simulink model "GolfSwing3D_SimscapePhysicalInterfaceSwitching"  (R2024b)
settings: Solver=VariableStepAuto  StartTime=0.0  StopTime=StopTime  MaxStep=0.001  RelTol=1e-3
model workspace: external: MAT-File 3DModelInputs.mat (data not in the file)
undefined symbols (not defined in the file): GripStrength, KillswitchFinalValue, KillswitchInitialValue, KillswitchStepTime, LeftLowerArmLength, PlaneTilt, RightLowerArmLength, UpperTorsoLength, X, Y, Z
libraries: nesl_utility x363, sm_lib x137, matrix_library x11, fl_lib x8, simulink x1
(part 10 of 13)

== system GolfSwing3D_SimscapePhysicalInterfaceSwitching/Left Elbow Joint/Revolute Joint/Subsystem ==
  note: Kinetic Enabled Subsystem
  Angular Velocity (rad/s) : Inport
  Enable : EnablePort
  Constant2 : Constant  Value=10
  Ideal Torque Sensor : fl_lib/Mechanical/Mechanical Sensors/Ideal Torque Sensor
  Ideal Torque Source : fl_lib/Mechanical/Mechanical Sources/Ideal Torque Source
  Mechanical Rotational Reference : fl_lib/Mechanical/Rotational Elements/Mechanical Rotational Reference
  PS-Simulink Converter : nesl_utility/PS-Simulink Converter  PhysicalDomain=network_engine_domain  SubClassName=ps_output  LeftPortType=input  RightPortType=output  PseudoPeriodic=off  Frequencies=[]  VectorFormat=inherit  Unit=inherit  AffineConversion=off
  Rotational Multibody Interface1 : fl_lib/Mechanical/Multibody Interfaces/Rotational Multibody Interface
  Simulink-PS Converter : nesl_utility/Simulink-PS Converter  PhysicalDomain=network_engine_domain  SubClassName=ps_input  LeftPortType=input  RightPortType=output  PseudoPeriodic=off  Frequencies=[]  NoiseDistribution=none  NoiseParameters=[]  Unit=rad/s  AffineConversion=off  FilteringAndDerivatives=provide  SimscapeFilterOrder=1  InputFilterTimeConstant=0.001  UdotUserProvided=0
  Simulink-PS Converter2 : nesl_utility/Simulink-PS Converter  PhysicalDomain=network_engine_domain  SubClassName=ps_input  LeftPortType=input  RightPortType=output  PseudoPeriodic=off  Frequencies=[]  NoiseDistribution=none  NoiseParameters=[]  Unit=1  AffineConversion=off  FilteringAndDerivatives=provide  SimscapeFilterOrder=1  InputFilterTimeConstant=0.001  UdotUserProvided=0
  Solver Configuration : nesl_utility/Solver Configuration  PhysicalDomain=network_engine_domain  SubClassName=solver  LeftPortType=input  RightPortType=generic  Tones=[]  Harmonics=[]  SimulateNoise=off  Profile=off  UseLocalSampling=off  EnableSwitchedLinearOptims=on  FrequencyDomain=off  UseCCode=off  RelTol=0.001  AbsTol=0.001  MinStep=1e-09  ToWorkspace=off  RevertToSquareIcSolve=off  NumHomotopyIterations=100  PhasorMode=off  PhasorModeNumHarmonics=1  ConsistencySolver=NEWTON_XTOL_AFTER_FTOL  IndexReductionMethod=DerivativeReplacement  DoDC=off  ResidualTolerance=1e-09  ConsistencyTolSource=GLOBAL  ConsistencyAbsTol=0.001  ConsistencyRelTol=0.001  ConsistencyTolFactor=0.001  UseLocalSolver=off  LocalSolverChoice=NE_BACKWARD_EULER_ADVANCER  ResolveIndetEquations=on  FunctionEvalNumThread=1  LocalSolverSampleTime=0.001  DoFixedCost=off  MaxNonlinIter=3  MaxModeIter=2  ComputeImpulses=off  ImpulseIterations=2  LinearAlgebra=auto  LinearAlgebraNumThread=0  EquationFormulation=NE_TIME_EF  DelaysMemoryBudget=1024  AutomaticFiltering=on  FilteringTimeConstant=0.001  PartitionStorageMethod=AS_NEEDED  PartitionMemoryBudget=1024  PartitionMethod=ROBUST  MultibodyUseLocalSolver=off  MultibodyLocalSolverChoice=ODE1  MultibodyLocalSolverSampleTime=0.001
  Torque (Nm) : Outport
  wires:
  Constant2/1 -> Simulink-PS Converter2/1
  PS-Simulink Converter/1 -> Torque (Nm)/1
  Angular Velocity (rad/s)/1 -> Simulink-PS Converter/1
  connections:
  Ideal Torque Sensor/RConn1 -- Rotational Multibody Interface1/RConn2
  Mechanical Rotational Reference/LConn1 -- Ideal Torque Source/RConn2 -- Solver Configuration/RConn1 -- Rotational Multibody Interface1/LConn2
  Rotational Multibody Interface1/LConn1 -- PS-Simulink Converter/LConn1
  Ideal Torque Source/LConn1 -- Ideal Torque Sensor/LConn1
  Simulink-PS Converter2/RConn1 -- Ideal Torque Source/RConn1
  Rotational Multibody Interface1/RConn1 -- Simulink-PS Converter/RConn1

== system GolfSwing3D_SimscapePhysicalInterfaceSwitching/Left Forearm/Left Forearm/LF Kinematically Driven ==
  Kinematically Driven LF : sm_lib/Joints/Revolute Joint  JointMode=Normal  CompositeWrenchDir=BaseOnFollower  CompositeWrenchFrame=FollowerFrame  SenseConstraintForce=off  SenseConstraintTorque=off  SenseTotalForce=off  SenseTotalTorque=on  PositionTargetSpecify=off  PositionTargetPriority=Low  PositionTargetValue=LFStartPosition  PositionTargetValueUnits=deg  VelocityTargetSpecify=off  VelocityTargetPriority=Low  VelocityTargetValue=LFStartVelocity  VelocityTargetValueUnits=deg/s  EquilibriumPosition=0  EquilibriumPositionUnits=deg  SpringStiffness=0  SpringStiffnessUnits=N*m/deg  DampingCoefficient=0  DampingCoefficientUnits=N*m/(deg/s)  LowerLimitSpecify=off  LowerLimitBound=0  LowerLimitBoundUnits=deg  LowerLimitStiffness=50  LowerLimitStiffnessUnits=N*m/deg  LowerLimitDamping=10  LowerLimitDampingUnits=N*m/(deg/s)  LowerLimitTransitionRegionWidth=0.1  LowerLimitTransitionRegionWidthUnits=deg  UpperLimitSpecify=off  UpperLimitBound=75  UpperLimitBoundUnits=deg  UpperLimitStiffness=50  UpperLimitStiffnessUnits=N*m/deg  UpperLimitDamping=10  UpperLimitDampingUnits=N*m/(deg/s)  UpperLimitTransitionRegionWidth=0.1  UpperLimitTransitionRegionWidthUnits=deg  TorqueActuationMode=ComputedTorque  MotionActuationMode=InputMotion  SensePosition=on  SenseVelocity=on  SenseAcceleration=off  SenseTorqueForce=on  SenseLowerLimitTorqueForce=off  SenseUpperLimitTorqueForce=off
  LFTorqueInput : nesl_utility/PS-Simulink Converter  PhysicalDomain=network_engine_domain  SubClassName=ps_output  LeftPortType=input  RightPortType=output  PseudoPeriodic=off  Frequencies=[]  VectorFormat=1-D array  Unit=inherit  AffineConversion=off
  PS-Simulink Converter : nesl_utility/PS-Simulink Converter  PhysicalDomain=network_engine_domain  SubClassName=ps_output  LeftPortType=input  RightPortType=output  PseudoPeriodic=off  Frequencies=[]  VectorFormat=1-D array  Unit=deg  AffineConversion=off
  PS-Simulink Converter1 : nesl_utility/PS-Simulink Converter  PhysicalDomain=network_engine_domain  SubClassName=ps_output  LeftPortType=input  RightPortType=output  PseudoPeriodic=off  Frequencies=[]  VectorFormat=1-D array  Unit=deg/s  AffineConversion=off
  PS-Simulink Converter2 : nesl_utility/PS-Simulink Converter  PhysicalDomain=network_engine_domain  SubClassName=ps_output  LeftPortType=input  RightPortType=output  PseudoPeriodic=off  Frequencies=[]  VectorFormat=1-D array  Unit=inherit  AffineConversion=off
  Simulink-PS Converter29 : nesl_utility/Simulink-PS Converter  PhysicalDomain=network_engine_domain  SubClassName=ps_input  LeftPortType=input  RightPortType=output  PseudoPeriodic=off  Frequencies=[]  NoiseDistribution=none  NoiseParameters=[]  Unit=deg  AffineConversion=off  FilteringAndDerivatives=provide  SimscapeFilterOrder=1  InputFilterTimeConstant=0.001  UdotUserProvided=2
  Bottom LF : PMIOPort  Side=Right
  Top LF : PMIOPort  Port=2  Side=Left
  tag scope: LFPosition=global, LFVelocity=global
  wires:
  [FcnOutLFPosition] -> Simulink-PS Converter29/1
  [FcnOutLFVelocity] -> Simulink-PS Converter29/2
  [FcnOutLFAcceleration] -> Simulink-PS Converter29/3
  PS-Simulink Converter/1 -> [LFPosition]  "LFPosition"
  PS-Simulink Converter1/1 -> [LFVelocity]  "LFVelocity"
  PS-Simulink Converter2/1 -> ?  "LFTorqueLocal"
  LFTorqueInput/1 -> ?  "LFTorqueInput"
  connections:
  Kinematically Driven LF/LConn1 -- Top LF/RConn1
  Kinematically Driven LF/RConn1 -- Bottom LF/RConn1
  Simulink-PS Converter29/RConn1 -- Kinematically Driven LF/LConn2
  PS-Simulink Converter1/LConn1 -- Kinematically Driven LF/RConn3
  PS-Simulink Converter2/LConn1 -- Kinematically Driven LF/RConn5
  PS-Simulink Converter/LConn1 -- Kinematically Driven LF/RConn2
  LFTorqueInput/LConn1 -- Kinematically Driven LF/RConn4

== system GolfSwing3D_SimscapePhysicalInterfaceSwitching/Left Forearm/Left Forearm/LF Kinetically Driven ==
  Kinetically Driven LF : sm_lib/Joints/Revolute Joint  JointMode=Normal  CompositeWrenchDir=BaseOnFollower  CompositeWrenchFrame=FollowerFrame  SenseConstraintForce=off  SenseConstraintTorque=off  SenseTotalForce=off  SenseTotalTorque=on  PositionTargetSpecify=on  PositionTargetPriority=Low  PositionTargetValue=LFStartPosition  PositionTargetValueUnits=deg  VelocityTargetSpecify=on  VelocityTargetPriority=Low  VelocityTargetValue=LFStartVelocity  VelocityTargetValueUnits=deg/s  EquilibriumPosition=0  EquilibriumPositionUnits=deg  SpringStiffness=0  SpringStiffnessUnits=N*m/deg  DampingCoefficient=0  DampingCoefficientUnits=N*m/(deg/s)  LowerLimitSpecify=off  LowerLimitBound=0  LowerLimitBoundUnits=deg  LowerLimitStiffness=50  LowerLimitStiffnessUnits=N*m/deg  LowerLimitDamping=10  LowerLimitDampingUnits=N*m/(deg/s)  LowerLimitTransitionRegionWidth=0.1  LowerLimitTransitionRegionWidthUnits=deg  UpperLimitSpecify=off  UpperLimitBound=75  UpperLimitBoundUnits=deg  UpperLimitStiffness=50  UpperLimitStiffnessUnits=N*m/deg  UpperLimitDamping=10  UpperLimitDampingUnits=N*m/(deg/s)  UpperLimitTransitionRegionWidth=0.1  UpperLimitTransitionRegionWidthUnits=deg  TorqueActuationMode=InputTorque  MotionActuationMode=ComputedMotion  SensePosition=on  SenseVelocity=on  SenseAcceleration=off  SenseTorqueForce=on  SenseLowerLimitTorqueForce=off  SenseUpperLimitTorqueForce=off
  LFTorque : nesl_utility/Simulink-PS Converter  PhysicalDomain=network_engine_domain  SubClassName=ps_input  LeftPortType=input  RightPortType=output  PseudoPeriodic=off  Frequencies=[]  NoiseDistribution=none  NoiseParameters=[]  Unit=N*m  AffineConversion=off  FilteringAndDerivatives=provide  SimscapeFilterOrder=1  InputFilterTimeConstant=0.001  UdotUserProvided=0
  LFTorqueInput : nesl_utility/PS-Simulink Converter  PhysicalDomain=network_engine_domain  SubClassName=ps_output  LeftPortType=input  RightPortType=output  PseudoPeriodic=off  Frequencies=[]  VectorFormat=1-D array  Unit=inherit  AffineConversion=off
  PS-Simulink Converter : nesl_utility/PS-Simulink Converter  PhysicalDomain=network_engine_domain  SubClassName=ps_output  LeftPortType=input  RightPortType=output  PseudoPeriodic=off  Frequencies=[]  VectorFormat=1-D array  Unit=deg  AffineConversion=off
  PS-Simulink Converter1 : nesl_utility/PS-Simulink Converter  PhysicalDomain=network_engine_domain  SubClassName=ps_output  LeftPortType=input  RightPortType=output  PseudoPeriodic=off  Frequencies=[]  VectorFormat=1-D array  Unit=deg/s  AffineConversion=off
  PS-Simulink Converter2 : nesl_utility/PS-Simulink Converter  PhysicalDomain=network_engine_domain  SubClassName=ps_output  LeftPortType=input  RightPortType=output  PseudoPeriodic=off  Frequencies=[]  VectorFormat=1-D array  Unit=inherit  AffineConversion=off
  Bottom LF : PMIOPort  Side=Right
  Top LF : PMIOPort  Port=2  Side=Left
  tag scope: LFPosition=global, LFVelocity=global
  wires:
  PS-Simulink Converter1/1 -> [LFVelocity]  "LFVelocity"
  PS-Simulink Converter/1 -> [LFPosition]  "LFPosition"
  [FcnOutLFTorque] -> LFTorque/1
  PS-Simulink Converter2/1 -> ?  "LFTorqueLocal"
  LFTorqueInput/1 -> ?  "LFTorqueInput"
  connections:
  Top LF/RConn1 -- Kinetically Driven LF/LConn1
  PS-Simulink Converter2/LConn1 -- Kinetically Driven LF/RConn5
  LFTorque/RConn1 -- Kinetically Driven LF/LConn2
  Kinetically Driven LF/RConn3 -- PS-Simulink Converter1/LConn1
  Kinetically Driven LF/RConn2 -- PS-Simulink Converter/LConn1
  Kinetically Driven LF/RConn1 -- Bottom LF/RConn1
  LFTorqueInput/LConn1 -- Kinetically Driven LF/RConn4

== system GolfSwing3D_SimscapePhysicalInterfaceSwitching/Right Forearm/Right Forearm/RF Kinematically Driven ==
  Kinematically Driven RF : sm_lib/Joints/Revolute Joint  JointMode=Normal  CompositeWrenchDir=BaseOnFollower  CompositeWrenchFrame=FollowerFrame  SenseConstraintForce=off  SenseConstraintTorque=off  SenseTotalForce=off  SenseTotalTorque=on  PositionTargetSpecify=off  PositionTargetPriority=Low  PositionTargetValue=RFStartPosition  PositionTargetValueUnits=deg  VelocityTargetSpecify=off  VelocityTargetPriority=Low  VelocityTargetValue=RFStartVelocity  VelocityTargetValueUnits=deg/s  EquilibriumPosition=0  EquilibriumPositionUnits=deg  SpringStiffness=0  SpringStiffnessUnits=N*m/deg  DampingCoefficient=0  DampingCoefficientUnits=N*m/(deg/s)  LowerLimitSpecify=off  LowerLimitBound=-15  LowerLimitBoundUnits=deg  LowerLimitStiffness=50  LowerLimitStiffnessUnits=N*m/deg  LowerLimitDamping=10  LowerLimitDampingUnits=N*m/(deg/s)  LowerLimitTransitionRegionWidth=0.1  LowerLimitTransitionRegionWidthUnits=deg  UpperLimitSpecify=off  UpperLimitBound=15  UpperLimitBoundUnits=deg  UpperLimitStiffness=50  UpperLimitStiffnessUnits=N*m/deg  UpperLimitDamping=10  UpperLimitDampingUnits=N*m/(deg/s)  UpperLimitTransitionRegionWidth=0.1  UpperLimitTransitionRegionWidthUnits=deg  TorqueActuationMode=ComputedTorque  MotionActuationMode=InputMotion  SensePosition=on  SenseVelocity=on  SenseAcceleration=off  SenseTorqueForce=on  SenseLowerLimitTorqueForce=off  SenseUpperLimitTorqueForce=off
  PS-Simulink Converter : nesl_utility/PS-Simulink Converter  PhysicalDomain=network_engine_domain  SubClassName=ps_output  LeftPortType=input  RightPortType=output  PseudoPeriodic=off  Frequencies=[]  VectorFormat=1-D array  Unit=deg  AffineConversion=off
  PS-Simulink Converter1 : nesl_utility/PS-Simulink Converter  PhysicalDomain=network_engine_domain  SubClassName=ps_output  LeftPortType=input  RightPortType=output  PseudoPeriodic=off  Frequencies=[]  VectorFormat=1-D array  Unit=deg/s  AffineConversion=off
  PS-Simulink Converter2 : nesl_utility/PS-Simulink Converter  PhysicalDomain=network_engine_domain  SubClassName=ps_output  LeftPortType=input  RightPortType=output  PseudoPeriodic=off  Frequencies=[]  VectorFormat=1-D array  Unit=inherit  AffineConversion=off
  RFTorqueInput : nesl_utility/PS-Simulink Converter  PhysicalDomain=network_engine_domain  SubClassName=ps_output  LeftPortType=input  RightPortType=output  PseudoPeriodic=off  Frequencies=[]  VectorFormat=1-D array  Unit=inherit  AffineConversion=off
  Simulink-PS Converter29 : nesl_utility/Simulink-PS Converter  PhysicalDomain=network_engine_domain  SubClassName=ps_input  LeftPortType=input  RightPortType=output  PseudoPeriodic=off  Frequencies=[]  NoiseDistribution=none  NoiseParameters=[]  Unit=deg  AffineConversion=off  FilteringAndDerivatives=provide  SimscapeFilterOrder=1  InputFilterTimeConstant=0.001  UdotUserProvided=2
  Conn1 : PMIOPort  Side=Right
  Conn5 : PMIOPort  Port=2  Side=Left
  tag scope: RFPosition=global, RFVelocity=global
  wires:
  [FcnOutRFVelocity] -> Simulink-PS Converter29/2
  [FcnOutRFPosition] -> Simulink-PS Converter29/1
  [FcnOutRFAcceleration] -> Simulink-PS Converter29/3
  PS-Simulink Converter/1 -> [RFPosition]  "RFPosition"
  PS-Simulink Converter1/1 -> [RFVelocity]  "RFVelocity"
  PS-Simulink Converter2/1 -> ?  "RFTorqueLocal"
  RFTorqueInput/1 -> ?  "RFTorqueInput"
  connections:
  Kinematically Driven RF/RConn1 -- Conn1/RConn1
  Simulink-PS Converter29/RConn1 -- Kinematically Driven RF/LConn2
  Kinematically Driven RF/LConn1 -- Conn5/RConn1
  PS-Simulink Converter/LConn1 -- Kinematically Driven RF/RConn2
  PS-Simulink Converter1/LConn1 -- Kinematically Driven RF/RConn3
  PS-Simulink Converter2/LConn1 -- Kinematically Driven RF/RConn5
  RFTorqueInput/LConn1 -- Kinematically Driven RF/RConn4

== system GolfSwing3D_SimscapePhysicalInterfaceSwitching/Right Forearm/Right Forearm/RF Kinetically Driven ==
  Kinetically Driven RF : sm_lib/Joints/Revolute Joint  JointMode=Normal  CompositeWrenchDir=BaseOnFollower  CompositeWrenchFrame=FollowerFrame  SenseConstraintForce=off  SenseConstraintTorque=off  SenseTotalForce=off  SenseTotalTorque=on  PositionTargetSpecify=on  PositionTargetPriority=Low  PositionTargetValue=RFStartPosition  PositionTargetValueUnits=deg  VelocityTargetSpecify=off  VelocityTargetPriority=Low  VelocityTargetValue=RFStartVelocity  VelocityTargetValueUnits=deg/s  EquilibriumPosition=0  EquilibriumPositionUnits=deg  SpringStiffness=0  SpringStiffnessUnits=N*m/deg  DampingCoefficient=0  DampingCoefficientUnits=N*m/(deg/s)  LowerLimitSpecify=off  LowerLimitBound=-15  LowerLimitBoundUnits=deg  LowerLimitStiffness=50  LowerLimitStiffnessUnits=N*m/deg  LowerLimitDamping=10  LowerLimitDampingUnits=N*m/(deg/s)  LowerLimitTransitionRegionWidth=0.1  LowerLimitTransitionRegionWidthUnits=deg  UpperLimitSpecify=off  UpperLimitBound=15  UpperLimitBoundUnits=deg  UpperLimitStiffness=50  UpperLimitStiffnessUnits=N*m/deg  UpperLimitDamping=10  UpperLimitDampingUnits=N*m/(deg/s)  UpperLimitTransitionRegionWidth=0.1  UpperLimitTransitionRegionWidthUnits=deg  TorqueActuationMode=InputTorque  MotionActuationMode=ComputedMotion  SensePosition=on  SenseVelocity=on  SenseAcceleration=off  SenseTorqueForce=on  SenseLowerLimitTorqueForce=off  SenseUpperLimitTorqueForce=off
  PS-Simulink Converter : nesl_utility/PS-Simulink Converter  PhysicalDomain=network_engine_domain  SubClassName=ps_output  LeftPortType=input  RightPortType=output  PseudoPeriodic=off  Frequencies=[]  VectorFormat=1-D array  Unit=deg  AffineConversion=off
  PS-Simulink Converter1 : nesl_utility/PS-Simulink Converter  PhysicalDomain=network_engine_domain  SubClassName=ps_output  LeftPortType=input  RightPortType=output  PseudoPeriodic=off  Frequencies=[]  VectorFormat=1-D array  Unit=deg/s  AffineConversion=off
  PS-Simulink Converter2 : nesl_utility/PS-Simulink Converter  PhysicalDomain=network_engine_domain  SubClassName=ps_output  LeftPortType=input  RightPortType=output  PseudoPeriodic=off  Frequencies=[]  VectorFormat=1-D array  Unit=inherit  AffineConversion=off
  RFTorque : nesl_utility/Simulink-PS Converter  PhysicalDomain=network_engine_domain  SubClassName=ps_input  LeftPortType=input  RightPortType=output  PseudoPeriodic=off  Frequencies=[]  NoiseDistribution=none  NoiseParameters=[]  Unit=N*m  AffineConversion=off  FilteringAndDerivatives=provide  SimscapeFilterOrder=1  InputFilterTimeConstant=0.001  UdotUserProvided=0
  RFTorqueInput : nesl_utility/PS-Simulink Converter  PhysicalDomain=network_engine_domain  SubClassName=ps_output  LeftPortType=input  RightPortType=output  PseudoPeriodic=off  Frequencies=[]  VectorFormat=1-D array  Unit=inherit  AffineConversion=off
  Conn1 : PMIOPort  Side=Right
  Conn2 : PMIOPort  Port=2  Side=Left
  tag scope: RFPosition=global, RFVelocity=global
  wires:
  PS-Simulink Converter1/1 -> [RFVelocity]  "RFVelocity"
  PS-Simulink Converter/1 -> [RFPosition]  "RFPosition"
  [FcnOutRFTorque] -> RFTorque/1
  PS-Simulink Converter2/1 -> ?  "RFTorqueLocal"
  RFTorqueInput/1 -> ?  "RFTorqueInput"
  connections:
  PS-Simulink Converter2/LConn1 -- Kinetically Driven RF/RConn5
  Kinetically Driven RF/RConn3 -- PS-Simulink Converter1/LConn1
  Conn1/RConn1 -- Kinetically Driven RF/RConn1
  Kinetically Driven RF/RConn2 -- PS-Simulink Converter/LConn1
  RFTorque/RConn1 -- Kinetically Driven RF/LConn2
  Conn2/RConn1 -- Kinetically Driven RF/LConn1
  RFTorqueInput/LConn1 -- Kinetically Driven RF/RConn4

== matlab function GolfSwing3D_SimscapePhysicalInterfaceSwitching/Spine Input Function/Spine Bending Torques ==
  data: Time input; Killswitch input; JointTorqueSpineX output; SpineInputXA parameter; SpineInputYA parameter; SpineInputXB parameter; SpineInputYB parameter; SpinePositionSetpointX parameter; GlobalGain parameter; JointTorqueSpineY output; SpineConstantX parameter; SpineConstantY parameter; SpineTimeGainX parameter; SpineTimeGainY parameter; SpineInputXC parameter; SpineInputYC parameter; SpinePositionGainX parameter; SpinePositionGainY parameter; TargetSpinePositionX parameter; TargetSpinePositionY parameter; TargetSpineVelocityX parameter; ModelingMode parameter; GlobalPCGain parameter; GlobalVCGain parameter; DampeningGlobalGain parameter; TargetImpactTime parameter; SpinePositionInputX output; SpinePositionInputY output; SpineVelocityInputX output; SpineVelocityInputY output; SpineAccelerationInputX output; SpineAccelerationInputY output; SpinePCGainX parameter; SpinePCGainY parameter; SpineAoX parameter; SpineAoY parameter; KinematicMode parameter; SpineDampeningX parameter; SpineDampeningY parameter; SpinePositionSetpointY parameter; SpineStartPositionX parameter; SpineStartPositionY parameter; SpineStartVelocityX parameter; SpineStartVelocityY parameter; SpineVCGainX parameter; SpineVCGainY parameter; SpinePositionX input; SpinePositionY input; SpineVelocityX input; SpineVelocityY input; TargetSpineVelocityY parameter; ZVCFSpineTorqueX parameter; ZVCFSpineTorqueY parameter; SpineAfX parameter; SpineAfY parameter; SpineInputXD parameter; SpineInputXE parameter; SpineInputXF parameter; SpineInputXG parameter; SpineInputYD parameter; SpineInputYE parameter; SpineInputYF parameter; SpineInputYG parameter
function [JointTorqueSpineX,JointTorqueSpineY,SpinePositionInputX,SpinePositionInputY,SpineVelocityInputX,...
    SpineVelocityInputY,SpineAccelerationInputX,SpineAccelerationInputY] = fcn(Time,Killswitch, SpineInputXA,SpineInputYA, SpineInputXB,SpineInputYB, SpinePositionSetpointX,GlobalGain,...
    SpineConstantX, SpineConstantY, SpineTimeGainX, SpineTimeGainY,...
    SpineInputXC, SpineInputYC, SpinePositionGainX, SpinePositionGainY,...
    TargetSpinePositionX, TargetSpinePositionY,TargetSpineVelocityX, ModelingMode,GlobalPCGain, GlobalVCGain,DampeningGlobalGain,TargetImpactTime,SpinePCGainX, SpinePCGainY, SpineAoX, SpineAoY, KinematicMode, SpineDampeningX, SpineDampeningY, SpinePositionSetpointY, SpineStartPositionX,...
    SpineStartPositionY, SpineStartVelocityX, SpineStartVelocityY, SpineVCGainX,...
    SpineVCGainY, SpinePositionX, SpinePositionY,SpineVelocityX, SpineVelocityY,...
    TargetSpineVelocityY, ZVCFSpineTorqueX, ZVCFSpineTorqueY,SpineAfX, SpineAfY,...
     SpineInputXD, SpineInputXE, SpineInputXF, SpineInputXG, SpineInputYD, SpineInputYE, SpineInputYF, SpineInputYG)

%Tau=Time/TargetImpactTime;
t=Time;

% %%%%%%%%%%%%%%%%%%%%%%%%%%%%%%%%%%%%%%%%%%%
% % Kinetic Input Selection and Calculation
% %%%%%%%%%%%%%%%%%%%%%%%%%%%%%%%%%%%%%%%%%%%

if ModelingMode==0
    % Values are all set to zero.
    JointTorqueSpineX=0;
    JointTorqueSpineY=0;
elseif ModelingMode==1
    % Control based strategy. Values are based on difference in value
    % between the current state and desired state.
    % Spine Joint Rotational Deltas
    DeltaSpinePositionX=SpinePositionX-TargetSpinePositionX;
    DeltaSpinePositionY=SpinePositionY-TargetSpinePositionY;
    DeltaSpineVelocityX=SpineVelocityX-TargetSpineVelocityX;
    DeltaSpineVelocityY=SpineVelocityY-TargetSpineVelocityY;
    % Control Based Strategy
    JointTorqueSpineX=DeltaSpinePositionX*SpinePCGainX*GlobalPCGain-DeltaSpineVelocityX*SpineVCGainX*GlobalVCGain-DampeningGlobalGain*SpineDampeningX*SpineVelocityX;
    JointTorqueSpineY=DeltaSpinePositionY*SpinePCGainY*GlobalPCGain-DeltaSpineVelocityY*SpineVCGainY*GlobalVCGain-DampeningGlobalGain*SpineDampeningY*SpineVelocityY;
elseif ModelingMode==2
    % Forward Dynamics Based Strategy. Values are computed based on a
    % polynomial and a combination of dampening and position gained
    % factors.
    JointTorqueSpineX=Killswitch*GlobalGain*(SpineConstantX+SpineTimeGainX*Time-SpinePositionGainX*(SpinePositionX-SpinePositionSetpointX)...
    -SpineDampeningX*SpineVelocityX);
    JointTorqueSpineY=Killswitch*GlobalGain*(SpineConstantY+SpineTimeGainY*Time-SpinePositionGainY*(SpinePositionY-SpinePositionSetpointY)...
    -SpineDampeningY*SpineVelocityY);
elseif ModelingMode==3
    JointTorqueSpineX=HexPolyInputFunction(SpineInputXA,SpineInputXB,SpineInputXC,SpineInputXD,SpineInputXE,SpineInputXF,SpineInputXG,Time)*Killswitch;
    JointTorqueSpineY=HexPolyInputFunction(SpineInputYA,SpineInputYB,SpineInputYC,SpineInputYD,SpineInputYE,SpineInputYF,SpineInputYG,Time)*Killswitch;
else
    %ZVCF Based Joint Torques. Values are pulled from model workspace and
    %held constant.
    JointTorqueSpineX=ZVCFSpineTorqueX;
    JointTorqueSpineY=ZVCFSpineTorqueY;
end

% %%%%%%%%%%%%%%%%%%%%%%%%%%%%%%%%%%%%%%%%%%%
% % Kinematic Input Selection and Calculation
% %%%%%%%%%%%%%%%%%%%%%%%%%%%%%%%%%%%%%%%%%%%

if KinematicMode==0
    % All kinematic values set to zero.
    SpinePositionInputX=0;
    SpinePositionInputY=0;
    SpineVelocityInputX=0;
    SpineVelocityInputY=0;
    SpineAccelerationInputX=0;
    SpineAccelerationInputY=0;
elseif KinematicMode==1
    % 1st Order Acceleration, 2nd Order Velocity, 3rd Order Position Solution
    PTX=TargetSpinePositionX;       
    VTX=TargetSpineVelocityX;
    PTY=TargetSpinePositionY;
    VTY=TargetSpineVelocityY;
    % Define Starting Position and Velocity
    PIX=SpineStartPositionX;
    VIX=SpineStartVelocityX;
    PIY=SpineStartPositionY;
    VIY=SpineStartVelocityY;
    AX=3*((VTX+VIX)*TargetImpactTime-2*(PTX-PIX))/TargetImpactTime^3;         % Constant in position equation
    BX=-2*((VTX+2*VIX)*TargetImpactTime-3*(PTX-PIX))/TargetImpactTime^2;         % Constant in position equation
    CX=VIX;         % Starting Velocity at Time Zero
    DX=PIX;         % Starting Position at Time Zero
    AY=3*((VTY+VIY)*TargetImpactTime-2*(PTY-PIY))/TargetImpactTime^3;         % Constant in position equation
    BY=-2*((VTY+2*VIY)*TargetImpactTime-3*(PTY-PIY))/TargetImpactTime^2;         % Constant in position equation
    CY=VIY;         % Starting Velocity at Time Zero
    DY=PIY;         % Starting Position at Time Zero
    % Equation for position as a function of time
    SpinePositionInputX=AX*Time^3/3+BX*Time^2/2+CX*Time+DX;
    SpinePositionInputY=AY*Time^3/3+BY*Time^2/2+CY*Time+DY;
    SpineVelocityInputX=AX*Time^2+BX*Time+CX;
    SpineVelocityInputY=AY*Time^2+BY*Time+CY;
    SpineAccelerationInputX=2*AX*Time+BX;
    SpineAccelerationInputY=2*AY*Time+BY;
elseif KinematicMode==2
    % 2nd Order Acceleration, 3rd Order Velocity, 4th Order Position Solution
    Tt=TargetImpactTime;
    t=Time;
    PoX=SpineStartPositionX;
    PoY=SpineStartPositionY;
    VoX=SpineStartVelocityX;
    VoY=SpineStartVelocityY;
    PfX=TargetSpinePositionX;
    PfY=TargetSpinePositionY;
    VfX=TargetSpineVelocityX;
    VfY=TargetSpineVelocityY;
    AoX=SpineAoX;
    AoY=SpineAoY;
    SpinePositionInputX=PoX + VoX*t + (AoX*t^2)/2 - (t^3*(4*PoX - 4*PfX + Tt*VfX + 3*Tt*VoX + AoX*Tt^2))/Tt^3 + (t^4*(6*PoX - 6*PfX + 2*Tt*VfX + 4*Tt*VoX + AoX*Tt^2))/(2*Tt^4);
    SpinePositionInputY=PoY + VoY*t + (AoY*t^2)/2 - (t^3*(4*PoY - 4*PfY + Tt*VfY + 3*Tt*VoY + AoY*Tt^2))/Tt^3 + (t^4*(6*PoY - 6*PfY + 2*Tt*VfY + 4*Tt*VoY + AoY*Tt^2))/(2*Tt^4);
    SpineVelocityInputX=VoX + AoX*t - (3*t^2*(4*PoX - 4*PfX + Tt*VfX + 3*Tt*VoX + AoX*Tt^2))/Tt^3 + (2*t^3*(6*PoX - 6*PfX + 2*Tt*VfX + 4*Tt*VoX + AoX*Tt^2))/Tt^4;
    SpineVelocityInputY=VoY + AoY*t - (3*t^2*(4*PoY - 4*PfY + Tt*VfY + 3*Tt*VoY + AoY*Tt^2))/Tt^3 + (2*t^3*(6*PoY - 6*PfY + 2*Tt*VfY + 4*Tt*VoY + AoY*Tt^2))/Tt^4;
    SpineAccelerationInputX=AoX + (6*t^2*(6*PoX - 6*PfX + 2*Tt*VfX + 4*Tt*VoX + AoX*Tt^2))/Tt^4 - (6*t*(4*PoX - 4*PfX + Tt*VfX + 3*Tt*VoX + AoX*Tt^2))/Tt^3;
    SpineAccelerationInputY=AoY + (6*t^2*(6*PoY - 6*PfY + 2*Tt*VfY + 4*Tt*VoY + AoY*Tt^2))/Tt^4 - (6*t*(4*PoY - 4*PfY + Tt*VfY + 3*Tt*VoY + AoY*Tt^2))/Tt^3;
else
    % 3rd Order Acceleration, 4th Order Velocity, 5th Order Position Solution
    Tt=TargetImpactTime;
    t=Time;
    PoX=SpineStartPositionX;
    PoY=SpineStartPositionY;
    VoX=SpineStartVelocityX;
    VoY=SpineStartVelocityY;
    PfX=TargetSpinePositionX;
    PfY=TargetSpinePositionY;
    VfX=TargetSpineVelocityX;
    VfY=TargetSpineVelocityY;
    AoX=SpineAoX;
    AoY=SpineAoY;
    AfX=SpineAfX;
    AfY=SpineAfY;
    SpinePositionInputX=PoX+VoX*t+(AoX*t^2)/2-(t^5*(12*PoX-12*PfX+6*Tt*VfX+6*Tt*VoX-AfX*Tt^2+AoX*Tt^2))/(2*Tt^5)-(t^3*(20*PoX-20*PfX+8*Tt*VfX+12*Tt*VoX-AfX*Tt^2+3*AoX*Tt^2))/(2*Tt^3)+(t^4*(30*PoX-30*PfX+14*Tt*VfX+16*Tt*VoX-2*AfX*Tt^2+3*AoX*Tt^2))/(2*Tt^4);
    SpinePositionInputY=PoY+VoY*t+(AoY*t^2)/2-(t^5*(12*PoY-12*PfY+6*Tt*VfY+6*Tt*VoY-AfY*Tt^2+AoY*Tt^2))/(2*Tt^5)-(t^3*(20*PoY-20*PfY+8*Tt*VfY+12*Tt*VoY-AfY*Tt^2+3*AoY*Tt^2))/(2*Tt^3)+(t^4*(30*PoY-30*PfY+14*Tt*VfY+16*Tt*VoY-2*AfY*Tt^2+3*AoY*Tt^2))/(2*Tt^4);  
    SpineVelocityInputX=VoX+AoX*t-(5*t^4*(12*PoX-12*PfX+6*Tt*VfX+6*Tt*VoX-AfX*Tt^2+AoX*Tt^2))/(2*Tt^5)-(3*t^2*(20*PoX-20*PfX+8*Tt*VfX+12*Tt*VoX-AfX*Tt^2+3*AoX*Tt^2))/(2*Tt^3)+(2*t^3*(30*PoX-30*PfX+14*Tt*VfX+16*Tt*VoX-2*AfX*Tt^2+3*AoX*Tt^2))/Tt^4;
    SpineVelocityInputY=VoY+AoY*t-(5*t^4*(12*PoY-12*PfY+6*Tt*VfY+6*Tt*VoY-AfY*Tt^2+AoY*Tt^2))/(2*Tt^5)-(3*t^2*(20*PoY-20*PfY+8*Tt*VfY+12*Tt*VoY-AfY*Tt^2+3*AoY*Tt^2))/(2*Tt^3)+(2*t^3*(30*PoY-30*PfY+14*Tt*VfY+16*Tt*VoY-2*AfY*Tt^2+3*AoY*Tt^2))/Tt^4;
    SpineAccelerationInputX=AoX-(3*t*(20*PoX-20*PfX+8*Tt*VfX+12*Tt*VoX-AfX*Tt^2+3*AoX*Tt^2))/Tt^3-(10*t^3*(12*PoX-12*PfX+6*Tt*VfX+6*Tt*VoX-AfX*Tt^2+AoX*Tt^2))/Tt^5+(6*t^2*(30*PoX-30*PfX+14*Tt*VfX+16*Tt*VoX-2*AfX*Tt^2+3*AoX*Tt^2))/Tt^4;
    SpineAccelerationInputY=AoY-(3*t*(20*PoY-20*PfY+8*Tt*VfY+12*Tt*VoY-AfY*Tt^2+3*AoY*Tt^2))/Tt^3-(10*t^3*(12*PoY-12*PfY+6*Tt*VfY+6*Tt*VoY-AfY*Tt^2+AoY*Tt^2))/Tt^5+(6*t^2*(30*PoY-30*PfY+14*Tt*VfY+16*Tt*VoY-2*AfY*Tt^2+3*AoY*Tt^2))/Tt^4;
end


% Calculate Higher Order Derivatives of the Position Outputs
SpineJerkX=gradient(SpineAccelerationInputX,t);
SpineJerkY=gradient(SpineAccelerationInputY,t);
SpineSnapX=gradient(SpineJerkX,t);
SpineSnapY=gradient(SpineJerkY,t);
SpineCrackleX=gradient(SpineSnapX,t);
SpineCrackleY=gradient(SpineSnapY,t);
SpinePopX=gradient(SpineCrackleX,t);
SpinePopY=gradient(SpineCrackleY,t);

== matlab function GolfSwing3D_SimscapePhysicalInterfaceSwitching/Hip Input Function/Hip Torque Output ==
  data: JointTorqueHipX output; Time input; Killswitch input; HipPositionX input; HipPositionY input; HipPositionZ input; HipVelocityX input; HipVelocityY input; HipVelocityZ input; HipInputXA parameter; HipInputYA parameter; HipInputZA parameter; HipInputXB parameter; HipInputYB parameter; HipInputZB parameter; HipPositionSetpointX parameter; HipPositionSetpointY parameter; GlobalGain parameter; JointTorqueHipY output; JointTorqueHipZ output; HipDampeningX parameter; HipDampeningY parameter; HipDampeningZ parameter; HipConstantX parameter; HipConstantY parameter; HipConstantZ parameter; HipTimeGainX parameter; HipTimeGainY parameter; HipTimeGainZ parameter; HipInputZC parameter; HipInputXC parameter; HipInputYC parameter; HipPositionGainX parameter; HipPositionGainY parameter; HipPositionGainZ parameter; HipPositionSetpointZ parameter; TargetHipPositionX parameter; TargetHipPositionY parameter; TargetHipPositionZ parameter; TargetHipVelocityX parameter; TargetHipVelocityY parameter; TargetHipVelocityZ parameter; HipPCGainX parameter; HipPCGainY parameter; HipPCGainZ parameter; HipVCGainX parameter; HipVCGainY parameter; HipVCGainZ parameter; ModelingMode parameter; ZVCFHipTorqueX parameter; ZVCFHipTorqueY parameter; ZVCFHipTorqueZ parameter; GlobalPCGain parameter; GlobalVCGain parameter; DampeningGlobalGain parameter; TargetImpactTime parameter; HipPositionInputX output; HipPositionInputY output; HipPositionInputZ output; HipVelocityInputX output; HipVelocityInputY output; HipVelocityInputZ output; HipAccelerationInputX output; HipAccelerationInputY output; HipAccelerationInputZ output; HipStartPositionX parameter; HipStartPositionY parameter; HipStartPositionZ parameter; HipStartVelocityX parameter; HipStartVelocityY parameter; HipStartVelocityZ parameter; KinematicMode parameter; HipAoX parameter; HipAoY parameter; HipAoZ parameter; HipAfX parameter; HipAfY parameter; HipAfZ parameter; HipInputXD parameter; HipInputYD parameter; HipInputXE parameter; HipInputXF parameter; HipInputXG parameter; HipInputYE parameter; HipInputYF parameter; HipInputYG parameter; HipInputZD parameter; HipInputZE parameter; HipInputZF parameter; HipInputZG parameter
function [JointTorqueHipX,JointTorqueHipY,JointTorqueHipZ,HipPositionInputX,HipPositionInputY,HipPositionInputZ,HipVelocityInputX,...
    HipVelocityInputY, HipVelocityInputZ,HipAccelerationInputX,HipAccelerationInputY,HipAccelerationInputZ] = fcn(Time,Killswitch, HipPositionX,HipPositionY,HipPositionZ, HipVelocityX,HipVelocityY,...
    HipVelocityZ,...
    HipInputXA,HipInputYA,HipInputZA, HipInputXB,HipInputYB,HipInputZB, HipPositionSetpointX,HipPositionSetpointY,GlobalGain,...
    HipDampeningX, HipDampeningY, HipDampeningZ, HipConstantX, HipConstantY, HipConstantZ, HipTimeGainX, HipTimeGainY, HipTimeGainZ, HipInputZC,...
    HipInputXC, HipInputYC, HipPositionGainX, HipPositionGainY, HipPositionGainZ, HipPositionSetpointZ,...
    TargetHipPositionX, TargetHipPositionY, TargetHipPositionZ, TargetHipVelocityX, TargetHipVelocityY, TargetHipVelocityZ,HipPCGainX, HipPCGainY, HipPCGainZ, HipVCGainX,...
    HipVCGainY, HipVCGainZ,ModelingMode,ZVCFHipTorqueX, ZVCFHipTorqueY, ZVCFHipTorqueZ,GlobalPCGain, GlobalVCGain,DampeningGlobalGain,TargetImpactTime,HipStartPositionX,...
    HipStartPositionY, HipStartPositionZ, HipStartVelocityX, HipStartVelocityY, HipStartVelocityZ,KinematicMode,HipAoX, HipAoY, HipAoZ,HipAfX, HipAfY, HipAfZ,...
    HipInputXD, HipInputYD, HipInputXE, HipInputXF, HipInputXG, HipInputYE, HipInputYF, HipInputYG, HipInputZD, HipInputZE, HipInputZF, HipInputZG)

%Tau=Time/TargetImpactTime;
t=Time;

% %%%%%%%%%%%%%%%%%%%%%%%%%%%%%%%%%%%%%%%%%%%
% % Kinetic Input Selection and Calculation
% %%%%%%%%%%%%%%%%%%%%%%%%%%%%%%%%%%%%%%%%%%%

if ModelingMode==0
    % Values are all set to zero.
    JointTorqueHipX=0;
    JointTorqueHipY=0;
    JointTorqueHipZ=0;
elseif ModelingMode==1
    % Control based strategy. Values are based on difference in value
    % between the current state and desired state.
    % Hip Joint Rotational Deltas
    DeltaHipPositionX=HipPositionX-TargetHipPositionX;
    DeltaHipPositionY=HipPositionY-TargetHipPositionY;
    DeltaHipPositionZ=HipPositionZ-TargetHipPositionZ;
    DeltaHipVelocityX=HipVelocityX-TargetHipVelocityX;
    DeltaHipVelocityY=HipVelocityY-TargetHipVelocityY;
    DeltaHipVelocityZ=HipVelocityZ-TargetHipVelocityZ;
    % Control Based Strategy
    JointTorqueHipX=DeltaHipPositionX*HipPCGainX*GlobalPCGain-DeltaHipVelocityX*HipVCGainX*GlobalVCGain-DampeningGlobalGain*HipDampeningX*HipVelocityX;
    JointTorqueHipY=DeltaHipPositionY*HipPCGainY*GlobalPCGain-DeltaHipVelocityY*HipVCGainY*GlobalVCGain-DampeningGlobalGain*HipDampeningY*HipVelocityY;
    JointTorqueHipZ=DeltaHipPositionZ*HipPCGainZ*GlobalPCGain-DeltaHipVelocityZ*HipVCGainZ*GlobalVCGain-DampeningGlobalGain*HipDampeningZ*HipVelocityZ;
elseif ModelingMode==2
    % Forward Dynamics Based Strategy. Values are computed based on a
    % polynomial and a combination of dampening and position gained
    % factors.
    JointTorqueHipX=Killswitch*GlobalGain*(HipConstantX+HipTimeGainX*Time-HipPositionGainX*(HipPositionX-HipPositionSetpointX)...
    -HipDampeningX*HipVelocityX);
    JointTorqueHipY=Killswitch*GlobalGain*(HipConstantY+HipTimeGainY*Time-HipPositionGainY*(HipPositionY-HipPositionSetpointY)...
    -HipDampeningY*HipVelocityY);
    JointTorqueHipZ=Killswitch*GlobalGain*(HipConstantZ+HipTimeGainZ*Time-HipPositionGainZ*(HipPositionZ-HipPositionSetpointZ)...
    -HipDampeningZ*HipVelocityZ);
elseif ModelingMode==3
    JointTorqueHipX=HexPolyInputFunction(HipInputXA,HipInputXB,HipInputXC,HipInputXD,HipInputXE,HipInputXF,HipInputXG,Time)*Killswitch;
    JointTorqueHipY=HexPolyInputFunction(HipInputYA,HipInputYB,HipInputYC,HipInputYD,HipInputYE,HipInputYF,HipInputYG,Time)*Killswitch;
    JointTorqueHipZ=HexPolyInputFunction(HipInputZA,HipInputZB,HipInputZC,HipInputZD,HipInputZE,HipInputZF,HipInputZG,Time)*Killswitch;
else
    %ZVCF Based Joint Torques. Values are pulled from model workspace and
    %held constant.
    JointTorqueHipX=ZVCFHipTorqueX;
    JointTorqueHipY=ZVCFHipTorqueY;
    JointTorqueHipZ=ZVCFHipTorqueZ;
end

% %%%%%%%%%%%%%%%%%%%%%%%%%%%%%%%%%%%%%%%%%%%
% % Kinematic Input Selection and Calculation
% %%%%%%%%%%%%%%%%%%%%%%%%%%%%%%%%%%%%%%%%%%%

if KinematicMode==0
    % All kinematic values set to zero.
    HipPositionInputX=0;
    HipPositionInputY=0;
    HipPositionInputZ=0;
    HipVelocityInputX=0;
    HipVelocityInputY=0;
    HipVelocityInputZ=0;
    HipAccelerationInputX=0;
    HipAccelerationInputY=0;
    HipAccelerationInputZ=0;
elseif KinematicMode==1
    % 1st Order Acceleration, 2nd Order Velocity, 3rd Order Position Solution
    PTX=TargetHipPositionX;       
    VTX=TargetHipVelocityX;
    PTY=TargetHipPositionY;
    VTY=TargetHipVelocityY;
    PTZ=TargetHipPositionZ;
    VTZ=TargetHipVelocityZ;
    % Define Starting Position and Velocity
    PIX=HipStartPositionX;
    VIX=HipStartVelocityX;
    PIY=HipStartPositionY;
    VIY=HipStartVelocityY;
    PIZ=HipStartPositionZ;
    VIZ=HipStartVelocityZ;
    AX=3*((VTX+VIX)*TargetImpactTime-2*(PTX-PIX))/TargetImpactTime^3;         % Constant in position equation
    BX=-2*((VTX+2*VIX)*TargetImpactTime-3*(PTX-PIX))/TargetImpactTime^2;         % Constant in position equation
    CX=VIX;         % Starting Velocity at Time Zero
    DX=PIX;         % Starting Position at Time Zero
    AY=3*((VTY+VIY)*TargetImpactTime-2*(PTY-PIY))/TargetImpactTime^3;         % Constant in position equation
    BY=-2*((VTY+2*VIY)*TargetImpactTime-3*(PTY-PIY))/TargetImpactTime^2;         % Constant in position equation
    CY=VIY;         % Starting Velocity at Time Zero
    DY=PIY;         % Starting Position at Time Zero
    AZ=3*((VTZ+VIZ)*TargetImpactTime-2*(PTZ-PIZ))/TargetImpactTime^3;         % Constant in position equation
    BZ=-2*((VTZ+2*VIZ)*TargetImpactTime-3*(PTZ-PIZ))/TargetImpactTime^2;         % Constant in position equation
    CZ=VIZ;         % Starting Velocity at Time Zero
    DZ=PIZ;         % Starting Position at Time Zero
    % Equation for position as a function of time
    HipPositionInputX=AX*Time^3/3+BX*Time^2/2+CX*Time+DX;
    HipPositionInputY=AY*Time^3/3+BY*Time^2/2+CY*Time+DY;
    HipPositionInputZ=AZ*Time^3/3+BZ*Time^2/2+CZ*Time+DZ;
    HipVelocityInputX=AX*Time^2+BX*Time+CX;
    HipVelocityInputY=AY*Time^2+BY*Time+CY;
    HipVelocityInputZ=AZ*Time^2+BZ*Time+CZ;
    HipAccelerationInputX=2*AX*Time+BX;
    HipAccelerationInputY=2*AY*Time+BY;
    HipAccelerationInputZ=2*AZ*Time+BZ;
elseif KinematicMode==2
    % 2nd Order Acceleration, 3rd Order Velocity, 4th Order Position Solution
    Tt=TargetImpactTime;
    t=Time;
    PoX=HipStartPositionX;
    PoY=HipStartPositionY;
    PoZ=HipStartPositionZ;
    VoX=HipStartVelocityX;
    VoY=HipStartVelocityY;
    VoZ=HipStartVelocityZ;
    PfX=TargetHipPositionX;
    PfY=TargetHipPositionY;
    PfZ=TargetHipPositionZ;
    VfX=TargetHipVelocityX;
    VfY=TargetHipVelocityY;
    VfZ=TargetHipVelocityZ;
    AoX=HipAoX;
    AoY=HipAoY;
    AoZ=HipAoZ;
    HipPositionInputX=PoX + VoX*t + (AoX*t^2)/2 - (t^3*(4*PoX - 4*PfX + Tt*VfX + 3*Tt*VoX + AoX*Tt^2))/Tt^3 + (t^4*(6*PoX - 6*PfX + 2*Tt*VfX + 4*Tt*VoX + AoX*Tt^2))/(2*Tt^4);
    HipPositionInputY=PoY + VoY*t + (AoY*t^2)/2 - (t^3*(4*PoY - 4*PfY + Tt*VfY + 3*Tt*VoY + AoY*Tt^2))/Tt^3 + (t^4*(6*PoY - 6*PfY + 2*Tt*VfY + 4*Tt*VoY + AoY*Tt^2))/(2*Tt^4);
    HipPositionInputZ=PoZ + VoZ*t + (AoZ*t^2)/2 - (t^3*(4*PoZ - 4*PfZ + Tt*VfZ + 3*Tt*VoZ + AoZ*Tt^2))/Tt^3 + (t^4*(6*PoZ - 6*PfZ + 2*Tt*VfZ + 4*Tt*VoZ + AoZ*Tt^2))/(2*Tt^4);
    HipVelocityInputX=VoX + AoX*t - (3*t^2*(4*PoX - 4*PfX + Tt*VfX + 3*Tt*VoX + AoX*Tt^2))/Tt^3 + (2*t^3*(6*PoX - 6*PfX + 2*Tt*VfX + 4*Tt*VoX + AoX*Tt^2))/Tt^4;
    HipVelocityInputY=VoY + AoY*t - (3*t^2*(4*PoY - 4*PfY + Tt*VfY + 3*Tt*VoY + AoY*Tt^2))/Tt^3 + (2*t^3*(6*PoY - 6*PfY + 2*Tt*VfY + 4*Tt*VoY + AoY*Tt^2))/Tt^4;
    HipVelocityInputZ=VoZ + AoZ*t - (3*t^2*(4*PoZ - 4*PfZ + Tt*VfZ + 3*Tt*VoZ + AoZ*Tt^2))/Tt^3 + (2*t^3*(6*PoZ - 6*PfZ + 2*Tt*VfZ + 4*Tt*VoZ + AoZ*Tt^2))/Tt^4;
    HipAccelerationInputX=AoX + (6*t^2*(6*PoX - 6*PfX + 2*Tt*VfX + 4*Tt*VoX + AoX*Tt^2))/Tt^4 - (6*t*(4*PoX - 4*PfX + Tt*VfX + 3*Tt*VoX + AoX*Tt^2))/Tt^3;
    HipAccelerationInputY=AoY + (6*t^2*(6*PoY - 6*PfY + 2*Tt*VfY + 4*Tt*VoY + AoY*Tt^2))/Tt^4 - (6*t*(4*PoY - 4*PfY + Tt*VfY + 3*Tt*VoY + AoY*Tt^2))/Tt^3;
    HipAccelerationInputZ=AoZ + (6*t^2*(6*PoZ - 6*PfZ + 2*Tt*VfZ + 4*Tt*VoZ + AoZ*Tt^2))/Tt^4 - (6*t*(4*PoZ - 4*PfZ + Tt*VfZ + 3*Tt*VoZ + AoZ*Tt^2))/Tt^3;
else
    % 3rd Order Acceleration, 4th Order Velocity, 5th Order Position Solution
    Tt=TargetImpactTime;
    t=Time;
    PoX=HipStartPositionX;
    PoY=HipStartPositionY;
    PoZ=HipStartPositionZ;
    VoX=HipStartVelocityX;
    VoY=HipStartVelocityY;
    VoZ=HipStartVelocityZ;
    PfX=TargetHipPositionX;
    PfY=TargetHipPositionY;
    PfZ=TargetHipPositionZ;
    VfX=TargetHipVelocityX;
    VfY=TargetHipVelocityY;
    VfZ=TargetHipVelocityZ;
    AoX=HipAoX;
    AoY=HipAoY;
    AoZ=HipAoZ;
    AfX=HipAfX;
    AfY=HipAfY;
    AfZ=HipAfZ;
    HipPositionInputX=PoX+VoX*t+(AoX*t^2)/2-(t^5*(12*PoX-12*PfX+6*Tt*VfX+6*Tt*VoX-AfX*Tt^2+AoX*Tt^2))/(2*Tt^5)-(t^3*(20*PoX-20*PfX+8*Tt*VfX+12*Tt*VoX-AfX*Tt^2+3*AoX*Tt^2))/(2*Tt^3)+(t^4*(30*PoX-30*PfX+14*Tt*VfX+16*Tt*VoX-2*AfX*Tt^2+3*AoX*Tt^2))/(2*Tt^4);
    HipPositionInputY=PoY+VoY*t+(AoY*t^2)/2-(t^5*(12*PoY-12*PfY+6*Tt*VfY+6*Tt*VoY-AfY*Tt^2+AoY*Tt^2))/(2*Tt^5)-(t^3*(20*PoY-20*PfY+8*Tt*VfY+12*Tt*VoY-AfY*Tt^2+3*AoY*Tt^2))/(2*Tt^3)+(t^4*(30*PoY-30*PfY+14*Tt*VfY+16*Tt*VoY-2*AfY*Tt^2+3*AoY*Tt^2))/(2*Tt^4);  
    HipPositionInputZ=PoZ+VoZ*t+(AoZ*t^2)/2-(t^5*(12*PoZ-12*PfZ+6*Tt*VfZ+6*Tt*VoZ-AfZ*Tt^2+AoZ*Tt^2))/(2*Tt^5)-(t^3*(20*PoZ-20*PfZ+8*Tt*VfZ+12*Tt*VoZ-AfZ*Tt^2+3*AoZ*Tt^2))/(2*Tt^3)+(t^4*(30*PoZ-30*PfZ+14*Tt*VfZ+16*Tt*VoZ-2*AfZ*Tt^2+3*AoZ*Tt^2))/(2*Tt^4);
    HipVelocityInputX=VoX+AoX*t-(5*t^4*(12*PoX-12*PfX+6*Tt*VfX+6*Tt*VoX-AfX*Tt^2+AoX*Tt^2))/(2*Tt^5)-(3*t^2*(20*PoX-20*PfX+8*Tt*VfX+12*Tt*VoX-AfX*Tt^2+3*AoX*Tt^2))/(2*Tt^3)+(2*t^3*(30*PoX-30*PfX+14*Tt*VfX+16*Tt*VoX-2*AfX*Tt^2+3*AoX*Tt^2))/Tt^4;
    HipVelocityInputY=VoY+AoY*t-(5*t^4*(12*PoY-12*PfY+6*Tt*VfY+6*Tt*VoY-AfY*Tt^2+AoY*Tt^2))/(2*Tt^5)-(3*t^2*(20*PoY-20*PfY+8*Tt*VfY+12*Tt*VoY-AfY*Tt^2+3*AoY*Tt^2))/(2*Tt^3)+(2*t^3*(30*PoY-30*PfY+14*Tt*VfY+16*Tt*VoY-2*AfY*Tt^2+3*AoY*Tt^2))/Tt^4;
    HipVelocityInputZ=VoZ+AoZ*t-(5*t^4*(12*PoZ-12*PfZ+6*Tt*VfZ+6*Tt*VoZ-AfZ*Tt^2+AoZ*Tt^2))/(2*Tt^5)-(3*t^2*(20*PoZ-20*PfZ+8*Tt*VfZ+12*Tt*VoZ-AfZ*Tt^2+3*AoZ*Tt^2))/(2*Tt^3)+(2*t^3*(30*PoZ-30*PfZ+14*Tt*VfZ+16*Tt*VoZ-2*AfZ*Tt^2+3*AoZ*Tt^2))/Tt^4;
    HipAccelerationInputX=AoX-(3*t*(20*PoX-20*PfX+8*Tt*VfX+12*Tt*VoX-AfX*Tt^2+3*AoX*Tt^2))/Tt^3-(10*t^3*(12*PoX-12*PfX+6*Tt*VfX+6*Tt*VoX-AfX*Tt^2+AoX*Tt^2))/Tt^5+(6*t^2*(30*PoX-30*PfX+14*Tt*VfX+16*Tt*VoX-2*AfX*Tt^2+3*AoX*Tt^2))/Tt^4;
    HipAccelerationInputY=AoY-(3*t*(20*PoY-20*PfY+8*Tt*VfY+12*Tt*VoY-AfY*Tt^2+3*AoY*Tt^2))/Tt^3-(10*t^3*(12*PoY-12*PfY+6*Tt*VfY+6*Tt*VoY-AfY*Tt^2+AoY*Tt^2))/Tt^5+(6*t^2*(30*PoY-30*PfY+14*Tt*VfY+16*Tt*VoY-2*AfY*Tt^2+3*AoY*Tt^2))/Tt^4;
    HipAccelerationInputZ=AoZ-(3*t*(20*PoZ-20*PfZ+8*Tt*VfZ+12*Tt*VoZ-AfZ*Tt^2+3*AoZ*Tt^2))/Tt^3-(10*t^3*(12*PoZ-12*PfZ+6*Tt*VfZ+6*Tt*VoZ-AfZ*Tt^2+AoZ*Tt^2))/Tt^5+(6*t^2*(30*PoZ-30*PfZ+14*Tt*VfZ+16*Tt*VoZ-2*AfZ*Tt^2+3*AoZ*Tt^2))/Tt^4;
end

% Calculate Higher Order Derivatives of the Position Outputs
HipJerkX=gradient(HipAccelerationInputX,t);
HipJerkY=gradient(HipAccelerationInputY,t);
HipJerkZ=gradient(HipAccelerationInputZ,t);
HipSnapX=gradient(HipJerkX,t);
HIpSnapY=gradient(HipJerkY,t);
HipSnapZ=gradient(HipJerkZ,t);
HipCrackleX=gradient(HipSnapX,t);
HipCrackleY=gradient(HIpSnapY,t);
HipCrackleZ=gradient(HipSnapZ,t);
HipPopX=gradient(HipCrackleX,t);
HipPopY=gradient(HipCrackleY,t);
HipPopZ=gradient(HipCrackleZ,t);

== matlab function GolfSwing3D_SimscapePhysicalInterfaceSwitching/Club Calculations/Subsystem/Total Wrist Forces and Torques Local ==
  data: LHTL input; RHTL input; LHTG input; RHTG input; LHFL input; RHFL input; LHFG input; RHFG input; HandPathVector input; MidpointVelocity input; TotalHandTorqueLocal output; TotalHandTorqueGlobal output; ClubTorqueMagnitude output; TotalHandForceLocal output; TotalHandForceGlobal output; ClubForceMagnitude output; HandForceYankLocal output; ForceAlongHandPath output; LinearPoweronClub output; LHAV input; RHAV input; LHonClubAngularPower output; RHonClubAngularPower output; LHMOF input; RHMOF input; SumofMomentsLHonClub output; SumofMomentsRHonClub output; LHVelocity input; RHVelocity input; LHandPathVector input; RHandPathVector input; LHonClubLinearPower output; RHonClubLinearPower output; LHForceAlongHandPath output; RHForceAlongHandPath output
function [TotalHandTorqueLocal,TotalHandTorqueGlobal,ClubTorqueMagnitude,TotalHandForceLocal,TotalHandForceGlobal,...
    ClubForceMagnitude,HandForceYankLocal,ForceAlongHandPath,LinearPoweronClub,...
    LHonClubAngularPower,RHonClubAngularPower,SumofMomentsLHonClub,SumofMomentsRHonClub,...
    LHonClubLinearPower,RHonClubLinearPower,LHForceAlongHandPath,RHForceAlongHandPath] = ...
    fcn(LHTL,RHTL,LHTG,RHTG,LHFL,RHFL,LHFG,RHFG,HandPathVector,MidpointVelocity,LHAV,RHAV,LHMOF,RHMOF,...
    LHVelocity,RHVelocity,LHandPathVector,RHandPathVector)

% Local Torques
TotalHandTorqueLocal = LHTL+RHTL;
ClubTorqueMagnitude=norm(TotalHandTorqueLocal);

% Local Forces
TotalHandForceLocal = LHFL+RHFL;
ClubForceMagnitude=norm(TotalHandForceLocal);
HandForceYankLocal=diff(TotalHandForceLocal);

% Global Torques
TotalHandTorqueGlobal=LHTG+RHTG;

% Global Forces
TotalHandForceGlobal=LHFG+RHFG;

% Force Along Hand Path
ForceAlongHandPath=dot(TotalHandForceGlobal,HandPathVector);
LHForceAlongHandPath=dot(LHFG,LHandPathVector);
RHForceAlongHandPath=dot(RHFG,RHandPathVector);

% Linear Power Applied to Club
LinearPoweronClub=dot(TotalHandForceGlobal,MidpointVelocity);
LHonClubLinearPower=dot(LHFG,LHVelocity);
RHonClubLinearPower=dot(RHFG,RHVelocity);

% Angular Power
LHonClubAngularPower=dot(LHTG,LHAV);
RHonClubAngularPower=dot(RHTG,RHAV);

% Sum of Moments
SumofMomentsLHonClub=LHMOF+LHTG;
SumofMomentsRHonClub=RHMOF+RHTG;
